simulink model "Model_Buildex_Subsystem_V4"  (R2021a)
settings: Solver=VariableStepAuto  StartTime=0.0  StopTime=10.0  RelTol=1e-3
settings Model: Creator=20204920  LastModifiedBy=20204920

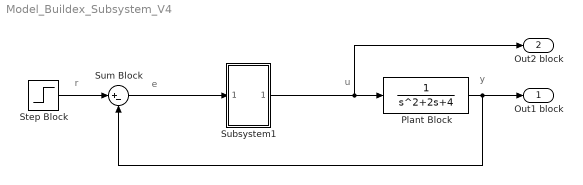
== system Model_Buildex_Subsystem_V4 ==
  note: y
  note: e
  note: u
  note: r
  Plant Block : TransferFcn  Denominator=[1 2 4]
  Step Block : Step  SampleTime=0
  Subsystem1 : Subsystem
  Sum Block : Sum  Inputs=|+-
  Out1 block : Outport
  Out2 block : Outport  Port=2
  wires:
  Plant Block/1 -> Out1 block/1, Sum Block/2
  Step Block/1 -> Sum Block/1
  Subsystem1/1(Out1) -> Plant Block/1, Out2 block/1
  Sum Block/1 -> Subsystem1/1(In1)

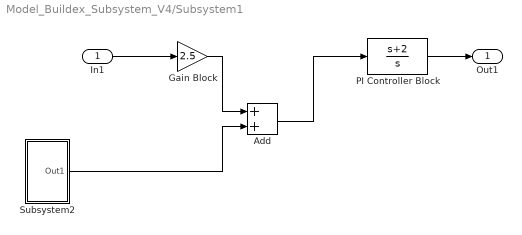
== system Model_Buildex_Subsystem_V4/Subsystem1 ==
  In1 : Inport
  Add : Sum
  Gain Block : Gain  Gain=2.5
  PI Controller Block : TransferFcn  Numerator=[1 2]  Denominator=[1 0]
  Subsystem2 : Subsystem
  Out1 : Outport
  wires:
  Gain Block/1 -> Add/1
  PI Controller Block/1 -> Out1/1
  In1/1 -> Gain Block/1
  Add/1 -> PI Controller Block/1
  Subsystem2/1(Out1) -> Add/2

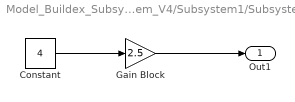
== system Model_Buildex_Subsystem_V4/Subsystem1/Subsystem2 ==
  Constant : Constant  Value=4
  Gain Block : Gain  Gain=2.5
  Out1 : Outport
  wires:
  Constant/1 -> Gain Block/1
  Gain Block/1 -> Out1/1
